simulink model "InvertedPendulumOpenLoop"  (Simulink 7.5)
settings: Solver=ode45  SolverMode=SingleTasking  StartTime=0.0  StopTime=2  RelTol=1e-3  AbsTol=1e-6
values from neighbouring files (symbols this model uses):
  b = 0.1    [IP_BODE.m]    (also in IP_DIS.m; IP_FDT.m; IP_PID_1.m; IP_PID_2.m)
  g = 9.8    [IP_BODE.m]    (also in IP_DIS.m; IP_FDT.m; IP_PID_1.m; IP_PID_2.m)
  i = 0.006    [IP_BODE.m]    (also in IP_DIS.m; IP_FDT.m; IP_PID_1.m; IP_PID_2.m)
  l = 0.3    [IP_BODE.m]    (also in IP_DIS.m; IP_FDT.m; IP_PID_1.m; IP_PID_2.m)
  M = .5    (= 0.5)    [IP_BODE.m]    (also in IP_DIS.m; IP_FDT.m; IP_PID_1.m; IP_PID_2.m)
  m = 0.2    [IP_BODE.m]    (also in IP_DIS.m; IP_FDT.m; IP_PID_1.m; IP_PID_2.m)
settings Model: Creator=neoben  LastModifiedBy=neoben
settings DataIOCC: LimitDataPoints=off
settings OptimizationCC: BlockReduction=off  BooleanDataType=off
settings DebuggingCC: SaveWithParameterizedLinksMsg=none  SignalResolutionControl=TryResolveAllWithWarning  SolverPrmCheckMsg=none  MultiTaskDSMMsg=warning  MultiTaskCondExecSysMsg=none  StrictBusMsg=None
settings HardwareCC: TargetUnknown=on
settings RTWCC: IncludeERTFirstTime=on

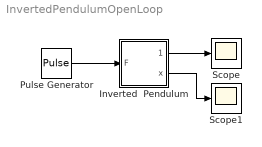
== system InvertedPendulumOpenLoop ==
  Inverted  Pendulum : Subsystem
  Pulse Generator : DiscretePulseGenerator  PulseType=Time based  Amplitude=1000  Period=10  PulseWidth=.01  PhaseDelay=0  SampleTime=1
  Scope : Scope
      settings: TickLabels=on  DataFormat=Array
  Scope1 : Scope
      settings: TickLabels=on  DataFormat=Array
  wires:
  Inverted  Pendulum/2(x) -> Scope1/1
  Inverted  Pendulum/1(Theta) -> Scope/1
  Pulse Generator/1 -> Inverted  Pendulum/1(F)

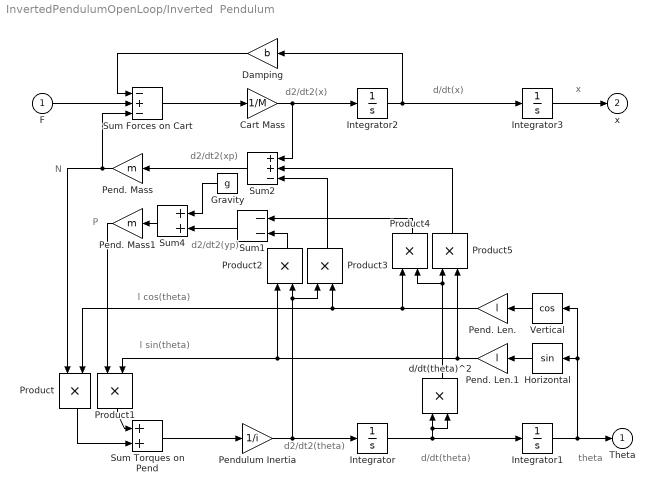
== system InvertedPendulumOpenLoop/Inverted  Pendulum ==
  note: theta
  note: d/dt(theta)
  note: d2/dt2(theta)
  note: d2/dt2(x)
  note: d/dt(x)
  note: x
  note: l cos(theta)
  note: l sin(theta)
  note: N
  note: P
  note: d2/dt2(yp)
  note: d2/dt2(xp)
  F : Inport
  Cart Mass : Gain  Gain=1/M  SaturateOnIntegerOverflow=on  OutDataTypeStr=Inherit: Same as input  ParamDataTypeStr=Inherit: Same as input
  Damping : Gain  Gain=b  SaturateOnIntegerOverflow=on  OutDataTypeStr=Inherit: Same as input  ParamDataTypeStr=Inherit: Same as input
  Gravity : Constant  Value=g
  Horizontal : Trigonometry
  Integrator{,1..3} (4 alike) : Integrator
  Pend. Len. : Gain  Gain=l  SaturateOnIntegerOverflow=on  OutDataTypeStr=Inherit: Same as input  ParamDataTypeStr=Inherit: Same as input
  Pend. Len.1 : Gain  Gain=l  SaturateOnIntegerOverflow=on  OutDataTypeStr=Inherit: Same as input  ParamDataTypeStr=Inherit: Same as input
  Pend. Mass : Gain  Gain=m  SaturateOnIntegerOverflow=on  OutDataTypeStr=Inherit: Same as input  ParamDataTypeStr=Inherit: Same as input
  Pend. Mass1 : Gain  Gain=m  SaturateOnIntegerOverflow=on  OutDataTypeStr=Inherit: Same as input  ParamDataTypeStr=Inherit: Same as input
  Pendulum Inertia : Gain  Gain=1/i  SaturateOnIntegerOverflow=on  OutDataTypeStr=Inherit: Same as input  ParamDataTypeStr=Inherit: Same as input
  Product{,1..5} (6 alike) : Product  SaturateOnIntegerOverflow=on  RndMeth=Zero  InputSameDT=on  OutDataTypeStr=Inherit: Same as first input
  Sum Forces on Cart : Sum  Inputs=-+-  SaturateOnIntegerOverflow=on  InputSameDT=on  OutDataTypeStr=Inherit: Same as first input
  Sum Torques on Pend : Sum  SaturateOnIntegerOverflow=on  InputSameDT=on  OutDataTypeStr=Inherit: Same as first input
  Sum1 : Sum  Inputs=--  SaturateOnIntegerOverflow=on  InputSameDT=on  OutDataTypeStr=Inherit: Same as first input
  Sum2 : Sum  Inputs=++-  SaturateOnIntegerOverflow=on  InputSameDT=on  OutDataTypeStr=Inherit: Same as first input
  Sum4 : Sum  SaturateOnIntegerOverflow=on  InputSameDT=on  OutDataTypeStr=Inherit: Same as first input
  Vertical : Trigonometry  Operator=cos
  d/dt(theta)^2 : Product  SaturateOnIntegerOverflow=on  RndMeth=Zero  InputSameDT=on  OutDataTypeStr=Inherit: Same as first input
  Theta : Outport
  x : Outport  Port=2
  wires:
  Integrator3/1 -> x/1
  Sum Forces on Cart/1 -> Cart Mass/1
  Sum Torques on Pend/1 -> Pendulum Inertia/1
  Integrator2/1 -> Integrator3/1, Damping/1
  Damping/1 -> Sum Forces on Cart/1
  F/1 -> Sum Forces on Cart/2
  Horizontal/1 -> Pend. Len.1/1
  Vertical/1 -> Pend. Len./1
  Integrator1/1 -> Theta/1, Horizontal/1, Vertical/1
  Product/1 -> Sum Torques on Pend/2
  Pend. Mass1/1 -> Product1/1
  Product1/1 -> Sum Torques on Pend/1
  Pend. Mass/1 -> Product/1, Sum Forces on Cart/3
  Gravity/1 -> Sum4/1
  Sum1/1 -> Sum4/2
  Sum4/1 -> Pend. Mass1/1
  Sum2/1 -> Pend. Mass/1
  Cart Mass/1 -> Integrator2/1, Sum2/1
  Pendulum Inertia/1 -> Integrator/1, Product3/1, Product2/2
  d/dt(theta)^2/1 -> Product5/1, Product4/2
  Pend. Len./1 -> Product/2, Product3/2, Product4/1
  Pend. Len.1/1 -> Product1/2, Product2/1, Product5/2
  Integrator/1 -> Integrator1/1, d/dt(theta)^2/1, d/dt(theta)^2/2
  Product5/1 -> Sum2/2
  Product4/1 -> Sum1/1
  Product3/1 -> Sum2/3
  Product2/1 -> Sum1/2
